simulink model "ssp5"  (R2014a)
settings: Solver=VariableStepDiscrete  StartTime=0.0  StopTime=20  RelTol=1e-3
libraries: dspvision x2, simulink x1
settings Model: Creator=root  LastModifiedBy=root

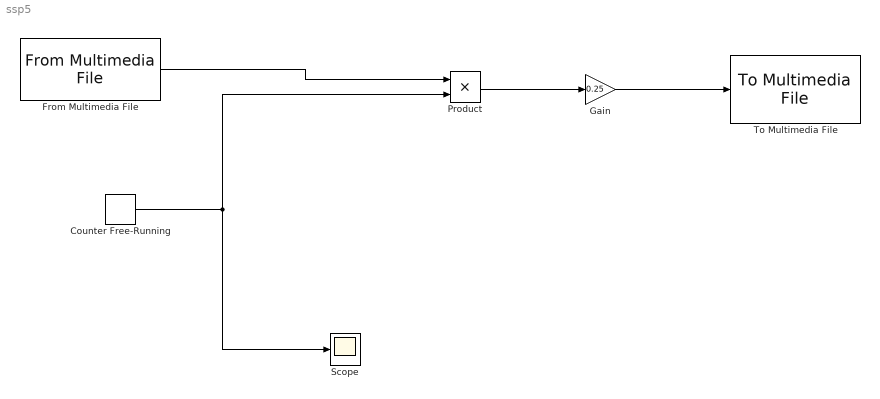
== system ssp5 ==
  Counter Free-Running : simulink/Sources/Counter Free-Running  NumBits=16  tsamp=-1
  From Multimedia File : dspvision/From Multimedia File  inputFilename=/home/brjathu/hawking01.wav  loop=on  numPlays=inf  outputStreams=Audio only  videoDataType=int16  audioDataType=int16  inheritSampleTime=on  userDefinedSampleTime=1/30  noAudioOutput=off  isIntensityVideo=off  fourcc=RGB  colorVideoFormat=One multidimensional signal  outputEOF=off  dataOrg=Column-major  audioFrameSize=1  computeAudioFrameSize=off  outSamplingMode=Sample based
  Gain : Gain  Gain=0.25  OutDataTypeStr=int32
  Product : Product
  Scope : Scope
  To Multimedia File : dspvision/To Multimedia File  outputFilename=output.wav  streamSelection=Audio only  videoCompressor=None (uncompressed)  audioCompressor=None (uncompressed)  imagePorts=One multidimensional signal  fileType=WAV  audioDatatype=Determine from input data type  fourcc=RGB  videoQuality=75  mj2000CompFactor=10
  wires:
  From Multimedia File/1 -> Product/1
  Product/1 -> Gain/1
  Gain/1 -> To Multimedia File/1
  Counter Free-Running/1 -> Scope/1, Product/2
